simulink model "CascadedControllerOnly"  (R2021a)
settings: Solver=VariableStepAuto  StartTime=0.0  StopTime=2  RelTol=1e-3
values from neighbouring files (symbols this model uses):
  A = lin_model.A    [linearize_boat.m]
  B = lin_model.B    [linearize_boat.m]
  C = lin_model.C    [linearize_boat.m]
  D = lin_model.D    [linearize_boat.m]
undefined symbols (not defined in the file or in its folder): ar2, br2, DiscIntNeverNeededParam
libraries: simulink x1, slctrlblks x1
settings Model: Creator=simao  LastModifiedBy=simao

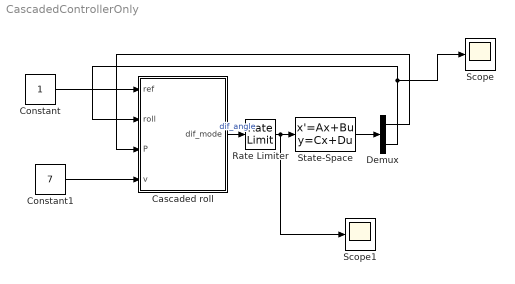
== system CascadedControllerOnly ==
  Cascaded roll : Subsystem  SystemSampleTime=0.02
  Constant : Constant
  Constant1 : Constant  Value=7
  Demux : Demux  Outputs=2
  Rate Limiter : RateLimiter  RisingSlewLimit=10  FallingSlewLimit=-10  SampleTimeMode=inherited
  Scope : Scope
  Scope1 : Scope
  State-Space : StateSpace  A=A  B=B  C=C  D=D  InitialCondition=0
  wires:
  Constant/1 -> Cascaded roll/1(ref)
  Constant1/1 -> Cascaded roll/4(v)
  State-Space/1 -> Demux/1
  Demux/1 -> Cascaded roll/3(P)
  Demux/2 -> Scope/1, Cascaded roll/2(roll)
  Cascaded roll/1(dif_mode) -> Rate Limiter/1  "dif_angle"
  Rate Limiter/1 -> Scope1/1, State-Space/1

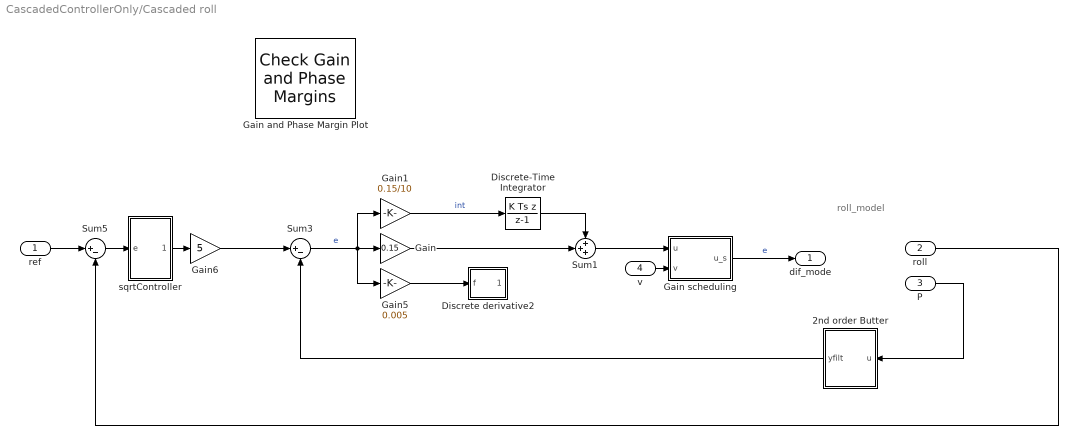
== system CascadedControllerOnly/Cascaded roll ==
  note: roll_model
  ref : Inport
  roll : Inport  Port=2
  P : Inport  Port=3
  v : Inport  Port=4
  2nd order Butter : Subsystem
  Discrete derivative2 : Subsystem
  Discrete-Time Integrator : DiscreteIntegrator  IntegratorMethod=Integration: Backward Euler  SampleTime=0.02  ICPrevOutput=DiscIntNeverNeededParam  ICPrevScaledInput=DiscIntNeverNeededParam
  Gain : Gain  Gain=0.15
  Gain and Phase Margin Plot : slctrlblks/Model Verification/Check Gain and Phase Margins  InstantiateOnLoad=on  SaveOperatingPoints=off  LinearizationIOs={'/Cascaded roll/Sum5', 1, 'in', 'off', '';'/Cascaded roll/roll', 1, 'out', 'on', ''}  LinearizeAt=SnapshotTimes  SnapshotTimes=[0]  TriggerType=rising  SampleTime=auto  RateConversionMethod=zoh  PreWarpFreq=10  UseExactDelayModel=off  UseFullBlockNameLabels=off  UseBusSignalLabels=off  enabled=on  stopWhenAssertionFail=off  export=off  ViewDlgPos=[1 41 1706.66666666667 954]  LaunchViewOnOpen=on  OpenViewOnLoad=off  FrequencyUnits=rad/s  MagnitudeUnits=dB  PhaseUnits=deg  TimeUnits=seconds  EnableMargins=off  GainMargin=[]  PhaseMargin=[]  PlotType=bode  FeedbackSign=-1
      settings: SourceProductBaseCode=SD  SaveToWorkspace=off  SaveName=sys
  Gain scheduling : MATLAB Function  TreatAsAtomicUnit=on
  Gain1 : Gain  Gain=0.15/10
  Gain5 : Gain  Gain=0.005
  Gain6 : Gain  Gain=5
  Sum1 : Sum  Inputs=+++
  Sum3 : Sum  Inputs=|+-
  Sum5 : Sum  Inputs=|+-
  sqrtController : Subsystem
  dif_mode : Outport  VectorParamsAs1DForOutWhenUnconnected=off
  wires:
  v/1 -> Gain scheduling/2(v)
  Gain6/1 -> Sum3/1
  Sum3/1 -> Gain1/1, Gain5/1, Gain/1  "e"
  Gain1/1 -> Discrete-Time Integrator/1  "int"
  Gain/1 -> Sum1/2
  ref/1 -> Sum5/1
  Sum1/1 -> Gain scheduling/1(u)
  Gain scheduling/1(u_s) -> dif_mode/1  "e"
  Discrete-Time Integrator/1 -> Sum1/1
  Sum5/1 -> sqrtController/1(e)
  sqrtController/1(Out1) -> Gain6/1
  roll/1 -> Sum5/2
  P/1 -> 2nd order Butter/1(u)
  Gain5/1 -> Discrete derivative2/1(f)
  2nd order Butter/1(yfilt) -> Sum3/2

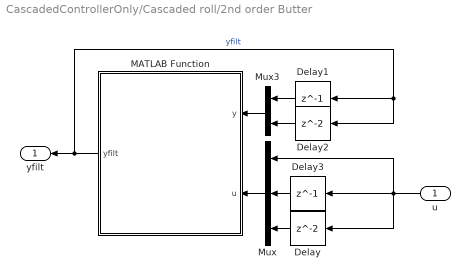
== system CascadedControllerOnly/Cascaded roll/2nd order Butter ==
  u : Inport
  Delay : Delay
  Delay1 : Delay  DelayLength=1  SampleTime=0.02
  Delay2 : Delay
  Delay3 : Delay  DelayLength=1  SampleTime=0.02
  MATLAB Function : MATLAB Function  TreatAsAtomicUnit=on
  Mux : Mux  Inputs=3
  Mux3 : Mux  Inputs=2
  yfilt : Outport
  wires:
  Mux3/1 -> MATLAB Function/1(y)
  Mux/1 -> MATLAB Function/2(u)
  MATLAB Function/1(yfilt) -> Delay1/1, Delay2/1, yfilt/1  "yfilt"
  Delay/1 -> Mux/3
  Delay3/1 -> Mux/2
  u/1 -> Mux/1, Delay3/1, Delay/1
  Delay1/1 -> Mux3/1
  Delay2/1 -> Mux3/2

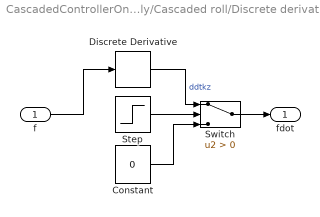
== system CascadedControllerOnly/Cascaded roll/Discrete derivative2 ==
  f : Inport
  Constant : Constant  Value=0
  Discrete Derivative : simulink/Discrete/Discrete Derivative  gainval=1.0  ICPrevScaledInput=0.0  OutMin=[]  OutMax=[]  OutDataType=fixdt(1, 16)  OutScaling=2^-10  DoSatur=off
  Step : Step  Time=0.01  Before=-1
  Switch : Switch  Criteria=u2 > Threshold
  fdot : Outport  VectorParamsAs1DForOutWhenUnconnected=off
  wires:
  Discrete Derivative/1 -> Switch/1  "ddtkz"
  Constant/1 -> Switch/3
  Step/1 -> Switch/2
  f/1 -> Discrete Derivative/1
  Switch/1 -> fdot/1

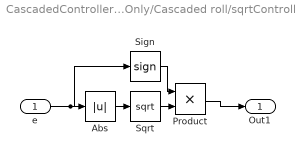
== system CascadedControllerOnly/Cascaded roll/sqrtController ==
  e : Inport
  Abs : Abs
  Product : Product
  Sign : Signum
  Sqrt : Sqrt  SaturateOnIntegerOverflow=on
  Out1 : Outport
  wires:
  Product/1 -> Out1/1
  e/1 -> Sign/1, Abs/1
  Abs/1 -> Sqrt/1
  Sqrt/1 -> Product/2
  Sign/1 -> Product/1

== matlab function CascadedControllerOnly/Cascaded roll/Gain scheduling ==
  data: u input; u_s output; v input
function u_s = fcn(u,v)
v_ref = 7;
if(v>v_ref)
    u_s = u*v_ref^2/v^2;
else
    u_s = u;
end

== matlab function CascadedControllerOnly/Cascaded roll/2nd order Butter/MATLAB Function ==
  data: y input; u input; yfilt output; br2 parameter; ar2 parameter
function yfilt = filtit(y,u, br2, ar2)
b = br2;
a = ar2;
yfilt = 0;
for i=1:length(u)
   yfilt = yfilt + b(i)*u(i);
end

for i=2:length(y)+1
   yfilt = yfilt - a(i)*y(i-1); 
end

yfilt = yfilt/a(1);

end
